simulink model "simulink16253801"  (R2018a)
settings: Solver=VariableStepAuto  StartTime=0.0  StopTime=50  RelTol=1e-3
libraries: powerlib x11
settings Model: Creator=pc_desktop  LastModifiedBy=pc_desktop

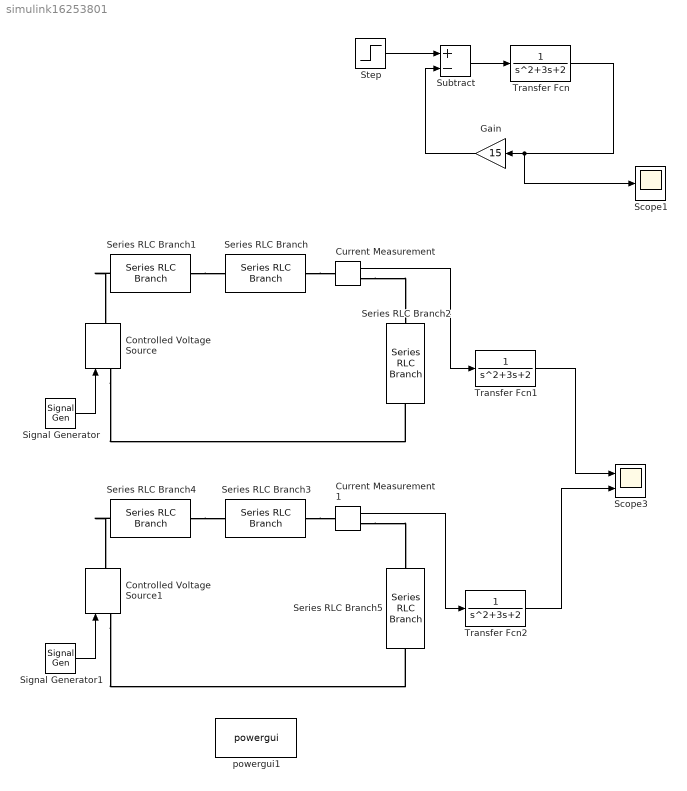
== system simulink16253801 ==
  Controlled Voltage Source : powerlib/Electrical Sources/Controlled Voltage Source  Tag=x(t)  Initialize=on  Source_Type=AC  Amplitude=0  Phase=0  Frequency=0  Measurements=None
      settings: AttributesFormatString=%<Tag>
  Controlled Voltage Source1 : powerlib/Electrical Sources/Controlled Voltage Source  Tag=x(t)  Initialize=on  Source_Type=AC  Amplitude=0  Phase=0  Frequency=0  Measurements=None
      settings: AttributesFormatString=%<Tag>
  Current Measurement : powerlib/Measurements/Current Measurement  PhasorSimulation=off  OutputType=Complex  PSBequivalent=0
  Current Measurement1 : powerlib/Measurements/Current Measurement  PhasorSimulation=off  OutputType=Complex  PSBequivalent=0
  Gain : Gain  Gain=15
  Scope1 : Scope
  Scope3 : Scope  NumInputPorts=2
  Series RLC Branch : powerlib/Elements/Series RLC Branch  LConnTagsString=__new0  RConnTagsString=__new0  BranchType=R  Resistance=3  Inductance=1e-3  SetiL0=off  InitialCurrent=0  Capacitance=1e-6  Setx0=off  InitialVoltage=0  Measurements=None
      settings: AttributesFormatString=%<Resistance> Ω
  Series RLC Branch1 : powerlib/Elements/Series RLC Branch  LConnTagsString=__new0  RConnTagsString=__new0  BranchType=L  Resistance=1  Inductance=1  SetiL0=off  InitialCurrent=0  Capacitance=1e-6  Setx0=off  InitialVoltage=0  Measurements=None
      settings: AttributesFormatString=%<Resistance> H
  Series RLC Branch2 : powerlib/Elements/Series RLC Branch  Tag=Vc(t)  LConnTagsString=__new0  RConnTagsString=__new0  BranchType=C  Resistance=1  Inductance=1e-3  SetiL0=off  InitialCurrent=0  Capacitance=0.5  Setx0=off  InitialVoltage=0  Measurements=None
      settings: AttributesFormatString=|
      | %<Capacitance> F
      | %<Tag>
  Series RLC Branch3 : powerlib/Elements/Series RLC Branch  LConnTagsString=__new0  RConnTagsString=__new0  BranchType=R  Resistance=4  Inductance=1e-3  SetiL0=off  InitialCurrent=0  Capacitance=1e-6  Setx0=off  InitialVoltage=0  Measurements=None
      settings: AttributesFormatString=%<Resistance> Ω
  Series RLC Branch4 : powerlib/Elements/Series RLC Branch  LConnTagsString=__new0  RConnTagsString=__new0  BranchType=L  Resistance=1  Inductance=1  SetiL0=off  InitialCurrent=0  Capacitance=1e-6  Setx0=off  InitialVoltage=0  Measurements=None
      settings: AttributesFormatString=%<Resistance> H
  Series RLC Branch5 : powerlib/Elements/Series RLC Branch  Tag=Vc(t)  LConnTagsString=__new0  RConnTagsString=__new0  BranchType=C  Resistance=1  Inductance=1e-3  SetiL0=off  InitialCurrent=0  Capacitance=0.0025  Setx0=off  InitialVoltage=0  Measurements=None
      settings: AttributesFormatString=|
      | %<Capacitance> F
      | %<Tag>
  Signal Generator : SignalGenerator  WaveForm=square  Frequency=500
  Signal Generator1 : SignalGenerator  WaveForm=square  Frequency=500
  Step : Step  After=15  SampleTime=0
  Subtract : Sum  Inputs=+-
  Transfer Fcn : TransferFcn  Denominator=[1 3 2]
  Transfer Fcn1 : TransferFcn  Denominator=[1 3 2]
  Transfer Fcn2 : TransferFcn  Denominator=[1 3 2]
  powergui1 : powerlib/powergui  Priority=1  SimulationMode=Continuous  SampleTime=50e-6  frequency=60  Iterations=50  frequencyindice=0  Pbase=100e6  ErrMax=1e-4  UnitsV=kV  UnitsW=MW  buscounter=0  FunctionMessages=off  echomessages=off  EnableUseOfTLC=off  CurrentSourceSwitches=off  DisableSnubberDevices=off  DisableRonSwitches=off  DisableVfSwitches=off  DisplayEquations=off  SolverType=Tustin/Backward Euler (TBE)  Interpol=off  ExternalGateDelay=off  methode=off  Ts=100  x0status=blocks  SPID=on  SwTol=0  HookPort=off  RestoreLinks=warning  ResistiveCurrentMeasurement=off  Frange=[0:2:500]  Ylog=off  Xlog=on  ShowGrid=off  save=off  variable=ZData  structure=0  ZoomFFT=off  StartTime=0.0  cycles=1  DisplayStyle=1  fundamental=60  FreqAxis=off  MaxFrequency=1000  frequencyindicesteady=1  RmsSteady=1  display=off
  wires:
  Signal Generator/1 -> Controlled Voltage Source/1
  Step/1 -> Subtract/1
  Subtract/1 -> Transfer Fcn/1
  Gain/1 -> Subtract/2
  Transfer Fcn/1 -> Scope1/1, Gain/1
  Transfer Fcn1/1 -> Scope3/1
  Transfer Fcn2/1 -> Scope3/2
  Signal Generator1/1 -> Controlled Voltage Source1/1
  Current Measurement/1 -> Transfer Fcn1/1
  Current Measurement1/1 -> Transfer Fcn2/1
  connections:
  Current Measurement/RConn1 -- Series RLC Branch2/LConn1
  Controlled Voltage Source/LConn1 -- Series RLC Branch2/RConn1
  Series RLC Branch1/LConn1 -- Series RLC Branch/RConn1
  Series RLC Branch1/RConn1 -- Controlled Voltage Source/RConn1
  Series RLC Branch/LConn1 -- Current Measurement/LConn1
  Controlled Voltage Source1/LConn1 -- Series RLC Branch5/RConn1
  Current Measurement1/RConn1 -- Series RLC Branch5/LConn1
  Series RLC Branch4/RConn1 -- Controlled Voltage Source1/RConn1
  Series RLC Branch3/LConn1 -- Current Measurement1/LConn1
  Series RLC Branch4/LConn1 -- Series RLC Branch3/RConn1
